simulink model "1"  (R2021a)
settings: Solver=VariableStepAuto  StartTime=0.0  StopTime=3  RelTol=1e-3
libraries: spsThreePhaseVIMeasurementLib x10, spsThreePhaseBreakerLib x9, spsThreePhaseSeriesRLCLoadLib x4, spsThreePhaseTransformerTwoWindingsLib x3, spsRMSLib x2, spsThreePhaseFaultLib x1, spsThreePhaseSourceLib x1, spspowerguiLib x1
settings Model: Creator=ranja  LastModifiedBy=vande

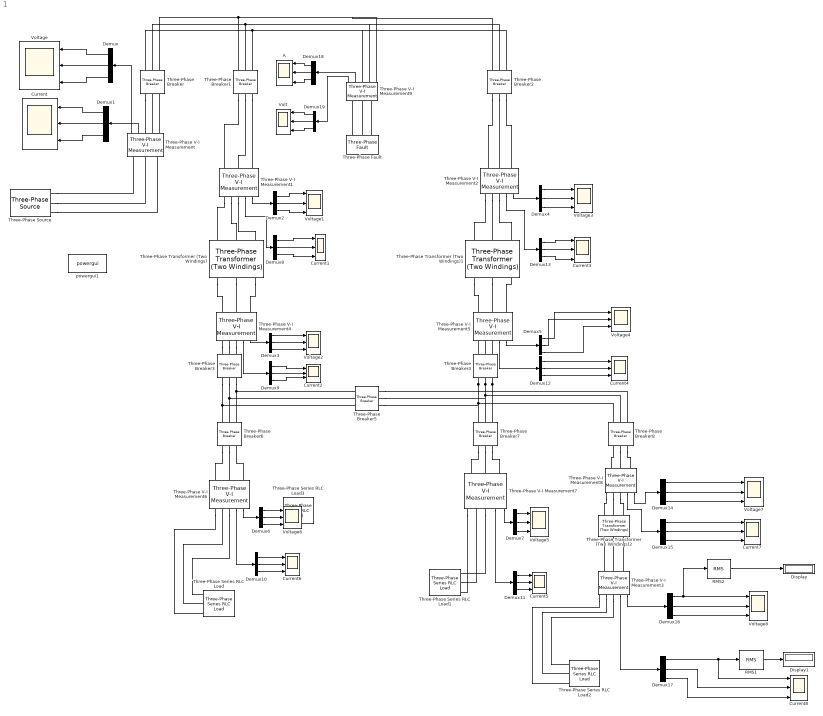
== system 1 ==
  A : Scope  NumInputPorts=3
  Current{,1..8} (9 alike) : Scope  NumInputPorts=3
  Demux{,1..19} (20 alike) : Demux  Outputs=3
  Display : Display
  Display1 : Display
  RMS1 : spsRMSLib/RMS  TrueRMS=on  Freq=50  RMSInit=0  Ts=0
  RMS2 : spsRMSLib/RMS  TrueRMS=on  Freq=50  RMSInit=0  Ts=0
  Three-Phase Series RLC Load : spsThreePhaseSeriesRLCLoadLib/Three-Phase Series RLC Load  LConnTagsString=A|B|C  Configuration=Y (grounded)  NominalVoltage=11e3  Vabc=[1e3 1e3 1e3]  Vabcp=[1e3 1e3 1e3]  NominalFrequency=50  UnbalancedPower=off  ActivePower=500e3  InductivePower=100  CapacitivePower=100  Pabc=[10e3 9e3 11e3]  QLabc=[100 90 110]  QCabc=[100 90 110]  Pabcp=[10e3 9e3 11e3]  QLabcp=[100 90 110]  QCabcp=[100 90 110]  Measurements=None  LoadType=constant Z
  Three-Phase Series RLC Load1 : spsThreePhaseSeriesRLCLoadLib/Three-Phase Series RLC Load  LConnTagsString=A|B|C  Configuration=Y (grounded)  NominalVoltage=11000  Vabc=[1e3 1e3 1e3]  Vabcp=[1e3 1e3 1e3]  NominalFrequency=50  UnbalancedPower=off  ActivePower=500e3  InductivePower=100  CapacitivePower=100  Pabc=[10e3 9e3 11e3]  QLabc=[100 90 110]  QCabc=[100 90 110]  Pabcp=[10e3 9e3 11e3]  QLabcp=[100 90 110]  QCabcp=[100 90 110]  Measurements=None  LoadType=constant Z
  Three-Phase Series RLC Load2 : spsThreePhaseSeriesRLCLoadLib/Three-Phase Series RLC Load  LConnTagsString=A|B|C  Configuration=Y (grounded)  NominalVoltage=433  Vabc=[1e3 1e3 1e3]  Vabcp=[1e3 1e3 1e3]  NominalFrequency=50  UnbalancedPower=off  ActivePower=10e3  InductivePower=5e3  CapacitivePower=10e3  Pabc=[10e3 9e3 11e3]  QLabc=[100 90 110]  QCabc=[100 90 110]  Pabcp=[10e3 9e3 11e3]  QLabcp=[100 90 110]  QCabcp=[100 90 110]  Measurements=None  LoadType=constant Z
  Three-Phase Series RLC Load3 : spsThreePhaseSeriesRLCLoadLib/Three-Phase Series RLC Load  LConnTagsString=A|B|C  Configuration=Y (grounded)  NominalVoltage=11000  Vabc=[1e3 1e3 1e3]  Vabcp=[1e3 1e3 1e3]  NominalFrequency=50  UnbalancedPower=off  ActivePower=500e3  InductivePower=100  CapacitivePower=100  Pabc=[10e3 9e3 11e3]  QLabc=[100 90 110]  QCabc=[100 90 110]  Pabcp=[10e3 9e3 11e3]  QLabcp=[100 90 110]  QCabcp=[100 90 110]  Measurements=None  LoadType=constant Z
  Three-Phase Transformer (Two Windings) : spsThreePhaseTransformerTwoWindingsLib/Three-Phase Transformer (Two Windings)  Winding1Connection=Yg  Winding2Connection=Yg  CoreType=Three single-phase transformers  SetSaturation=off  Hysteresis=off  DataFile='hysteresis'  SetInitialFlux=off  Measurements=None  UNITS=pu  NominalPower=[ 2000e3 , 50 ]  Winding1=[ 33e3 , 0.002 , 0.08 ]  Winding2=[ 11e3 , 0.002 , 0.08 ]  Rm=500  Lm=500  L0=0.5  Saturation=[ 0,0 ; 0.0024,1.2 ; 1.0,1.52 ]  InitialFluxes=[ 0.8 , -0.8 , 0.7 ]  BreakLoop=off  DiscreteSolver=Trapezoidal iterative  DataType=off  TransfoNumber=1
  Three-Phase Transformer (Two Windings)1 : spsThreePhaseTransformerTwoWindingsLib/Three-Phase Transformer (Two Windings)  Winding1Connection=Yg  Winding2Connection=Yg  CoreType=Three single-phase transformers  SetSaturation=off  Hysteresis=off  DataFile='hysteresis'  SetInitialFlux=off  Measurements=None  UNITS=pu  NominalPower=[ 2000e3 , 50 ]  Winding1=[ 33e3 , 0.002 , 0.08 ]  Winding2=[ 11e3 , 0.002 , 0.08 ]  Rm=500  Lm=500  L0=0.5  Saturation=[ 0,0 ; 0.0024,1.2 ; 1.0,1.52 ]  InitialFluxes=[ 0.8 , -0.8 , 0.7 ]  BreakLoop=off  DiscreteSolver=Trapezoidal iterative  DataType=off  TransfoNumber=1
  Three-Phase Transformer (Two Windings)2 : spsThreePhaseTransformerTwoWindingsLib/Three-Phase Transformer (Two Windings)  Winding1Connection=Yg  Winding2Connection=Yg  CoreType=Three single-phase transformers  SetSaturation=off  Hysteresis=off  DataFile='hysteresis'  SetInitialFlux=off  Measurements=None  UNITS=pu  NominalPower=[ 500e3 , 50 ]  Winding1=[ 11e3 , 0.002 , 0.08 ]  Winding2=[ 0.433e3 , 0.002 , 0.08 ]  Rm=500  Lm=500  L0=0.5  Saturation=[ 0,0 ; 0.0024,1.2 ; 1.0,1.52 ]  InitialFluxes=[ 0.8 , -0.8 , 0.7 ]  BreakLoop=off  DiscreteSolver=Trapezoidal iterative  DataType=off  TransfoNumber=1
  Three-Phase V-I Measurement{,1..9} (10 alike) : spsThreePhaseVIMeasurementLib/Three-Phase V-I Measurement  VoltageMeasurement=phase-to-ground  SetLabelV=off  LabelV=Vabc  Vpu=off  VpuLL=off  CurrentMeasurement=yes  SetLabelI=off  LabelI=Iabc  Ipu=off  Pbase=100e6  Vbase=500e3  OutputType=Complex  PhasorSimulation=off  PSBequivalent=0
  Three-Phase Breaker{,1..8} (9 alike) : spsThreePhaseBreakerLib/Three-Phase Breaker  InitialState=closed  SwitchA=on  SwitchB=on  SwitchC=on  SwitchTimes="[1/60  5/60]"  External=off  BreakerResistance=0.01  SnubberResistance=1e6  SnubberCapacitance=inf  Measurements=None
  Three-Phase Fault : spsThreePhaseFaultLib/Three-Phase Fault  InitialStates=0  FaultA=on  FaultB=on  FaultC=on  GroundFault=on  SwitchTimes=[1 1.5]  External=off  SwitchStatus=NaN  FaultResistance=17  GroundResistance=0.01  SnubberResistance=1e6  SnubberCapacitance=inf  Measurements=None
  Three-Phase Source : spsThreePhaseSourceLib/Three-Phase Source  InternalConnection=Yg  VoltagePhases=off  Voltage=33e3  PhaseAngle=0  Voltage_phases=[25e3 25e3 25e3]/sqrt(3)  PhaseAngles_phases=[0 -120 +120]  Frequency=50  NonIdealSource=on  SpecifyImpedance=off  Resistance=0.8929  Inductance=16.58e-3  ShortCircuitLevel=100e6  BaseVoltage=25e3  XRratio=7  BusType=swing  Pref=10e3  Qref=0  Prefabc=[10e3, 10e3, 10e3]  Qrefabc=[0, 0, 0]  Qmin=-inf  Qmax=inf
  Volt : Scope  NumInputPorts=3
  Voltage{,1..8} (9 alike) : Scope  NumInputPorts=3
  powergui1 : spspowerguiLib/powergui  Priority=1  SimulationMode=Discrete  SampleTime=1e-4  frequency=60  Iterations=50  frequencyindice=0  Pbase=100e6  ErrMax=1e-4  UnitsV=kV  UnitsW=MW  buscounter=0  FunctionMessages=off  echomessages=off  EnableUseOfTLC=off  CurrentSourceSwitches=off  DisableSnubberDevices=off  DisableRonSwitches=off  DisableVfSwitches=off  DisplayEquations=off  AutomaticDiscreteSolvers=off  SolverType=Tustin/Backward Euler (TBE)  Interpol=off  ExternalGateDelay=off  methode=off  Ts=100  x0status=blocks  SPID=on  SwTol=0  HookPort=off  NonlinearTolerance=1e-4  nMaxIteration=100  ContinueOnMaxIteration=off  RestoreLinks=warning  ResistiveCurrentMeasurement=off  Frange=[0:2:500]  Ylog=off  Xlog=on  ShowGrid=off  save=off  variable=ZData  structure=0  ZoomFFT=off  StartTime=0.0  cycles=1  DisplayStyle=1  fundamental=60  FreqAxis=off  MaxFrequency=1000  frequencyindicesteady=1  RmsSteady=1  display=off
  wires:
  Three-Phase V-I Measurement/2 -> Demux1/1
  Demux/1 -> Voltage/1
  Demux/3 -> Voltage/3
  Demux/2 -> Voltage/2
  Demux13/3 -> Current3/3
  Demux16/1 -> Voltage8/1, RMS2/1
  Demux1/3 -> Current/3
  Demux16/3 -> Voltage8/3
  RMS1/1 -> Display1/1
  Three-Phase V-I Measurement5/2 -> Demux12/1
  Demux17/3 -> Current8/3
  Demux9/1 -> Current2/1
  Three-Phase V-I Measurement3/1 -> Demux16/1
  Demux17/2 -> Current8/2
  RMS2/1 -> Display/1
  Demux15/2 -> Current7/2
  Three-Phase V-I Measurement/1 -> Demux/1
  Demux14/2 -> Voltage7/2
  Three-Phase V-I Measurement8/1 -> Demux14/1
  Three-Phase V-I Measurement8/2 -> Demux15/1
  Three-Phase V-I Measurement2/2 -> Demux13/1
  Three-Phase V-I Measurement3/2 -> Demux17/1
  Demux13/2 -> Current3/2
  Three-Phase V-I Measurement7/2 -> Demux11/1
  Three-Phase V-I Measurement5/1 -> Demux5/1
  Demux4/3 -> Voltage3/3
  Demux4/2 -> Voltage3/2
  Three-Phase V-I Measurement2/1 -> Demux4/1
  Demux3/3 -> Voltage2/3
  Demux2/2 -> Voltage1/2
  Demux14/1 -> Voltage7/1
  Demux2/1 -> Voltage1/1
  Demux1/2 -> Current/2
  Demux2/3 -> Voltage1/3
  Demux13/1 -> Current3/1
  Demux12/3 -> Current4/3
  Three-Phase V-I Measurement1/1 -> Demux2/1
  Demux11/2 -> Current5/2
  Demux10/3 -> Current6/3
  Demux12/1 -> Current4/1
  Three-Phase V-I Measurement6/2 -> Demux10/1
  Demux11/3 -> Current5/3
  Demux3/1 -> Voltage2/1
  Demux9/3 -> Current2/3
  Demux15/3 -> Current7/3
  Demux10/1 -> Current6/1
  Demux3/2 -> Voltage2/2
  Three-Phase V-I Measurement6/1 -> Demux6/1
  Demux5/2 -> Voltage4/2
  Three-Phase V-I Measurement7/1 -> Demux7/1
  Demux9/2 -> Current2/2
  Demux7/2 -> Voltage5/2
  Demux7/1 -> Voltage5/1
  Demux8/2 -> Current1/2
  Demux11/1 -> Current5/1
  Demux5/3 -> Voltage4/3
  Demux14/3 -> Voltage7/3
  Demux5/1 -> Voltage4/1
  Demux8/3 -> Current1/3
  Demux6/2 -> Voltage6/2
  Demux17/1 -> RMS1/1, Current8/1
  Demux1/1 -> Current/1
  Demux16/2 -> Voltage8/2
  Demux15/1 -> Current7/1
  Demux12/2 -> Current4/2
  Demux4/1 -> Voltage3/1
  Demux7/3 -> Voltage5/3
  Demux6/3 -> Voltage6/3
  Three-Phase V-I Measurement4/2 -> Demux9/1
  Demux10/2 -> Current6/2
  Three-Phase V-I Measurement1/2 -> Demux8/1
  Demux6/1 -> Voltage6/1
  Demux8/1 -> Current1/1
  Three-Phase V-I Measurement4/1 -> Demux3/1
  Three-Phase V-I Measurement9/1 -> Demux19/1
  Three-Phase V-I Measurement9/2 -> Demux18/1
  Demux18/2 -> A/2
  Demux18/1 -> A/1
  Demux18/3 -> A/3
  Demux19/1 -> Volt/1
  Demux19/2 -> Volt/2
  Demux19/3 -> Volt/3
  connections:
  Three-Phase Breaker3/RConn3 -- Three-Phase Breaker5/LConn3 -- Three-Phase Breaker6/LConn3
  Three-Phase Breaker4/RConn2 -- Three-Phase Breaker5/RConn2 -- Three-Phase Breaker7/LConn2 -- Three-Phase Breaker8/LConn2
  Three-Phase Breaker1/LConn3 -- Three-Phase V-I Measurement9/RConn3 -- Three-Phase Breaker2/LConn3 -- Three-Phase Breaker/RConn3
  Three-Phase Breaker3/RConn2 -- Three-Phase Breaker5/LConn2 -- Three-Phase Breaker6/LConn2
  Three-Phase Breaker4/RConn3 -- Three-Phase Breaker5/RConn3 -- Three-Phase Breaker7/LConn3 -- Three-Phase Breaker8/LConn3
  Three-Phase Breaker1/LConn1 -- Three-Phase V-I Measurement9/RConn1 -- Three-Phase Breaker2/LConn1 -- Three-Phase Breaker/RConn1
  Three-Phase Breaker4/RConn1 -- Three-Phase Breaker5/RConn1 -- Three-Phase Breaker8/LConn1 -- Three-Phase Breaker7/LConn1
  Three-Phase Breaker3/RConn1 -- Three-Phase Breaker5/LConn1 -- Three-Phase Breaker6/LConn1
  Three-Phase Breaker1/LConn2 -- Three-Phase V-I Measurement9/RConn2 -- Three-Phase Breaker2/LConn2 -- Three-Phase Breaker/RConn2
  Three-Phase Source/RConn1 -- Three-Phase V-I Measurement/LConn1
  Three-Phase V-I Measurement4/RConn2 -- Three-Phase Breaker3/LConn2
  Three-Phase V-I Measurement/RConn3 -- Three-Phase Breaker/LConn3
  Three-Phase Breaker/LConn1 -- Three-Phase V-I Measurement/RConn1
  Three-Phase V-I Measurement3/RConn1 -- Three-Phase Series RLC Load2/LConn1
  Three-Phase V-I Measurement8/RConn3 -- Three-Phase Transformer (Two Windings)2/LConn3
  Three-Phase Source/RConn3 -- Three-Phase V-I Measurement/LConn3
  Three-Phase Breaker7/RConn3 -- Three-Phase V-I Measurement7/LConn3
  Three-Phase V-I Measurement8/LConn3 -- Three-Phase Breaker8/RConn3
  Three-Phase Breaker2/RConn3 -- Three-Phase V-I Measurement2/LConn3
  Three-Phase Breaker2/RConn1 -- Three-Phase V-I Measurement2/LConn1
  Three-Phase V-I Measurement6/LConn1 -- Three-Phase Breaker6/RConn1
  Three-Phase V-I Measurement1/RConn2 -- Three-Phase Transformer (Two Windings)/LConn2
  Three-Phase Breaker8/RConn2 -- Three-Phase V-I Measurement8/LConn2
  Three-Phase Transformer (Two Windings)/RConn2 -- Three-Phase V-I Measurement4/LConn2
  Three-Phase V-I Measurement2/RConn2 -- Three-Phase Transformer (Two Windings)1/LConn2
  Three-Phase Breaker2/RConn2 -- Three-Phase V-I Measurement2/LConn2
  Three-Phase V-I Measurement3/RConn3 -- Three-Phase Series RLC Load2/LConn3
  Three-Phase V-I Measurement4/RConn3 -- Three-Phase Breaker3/LConn3
  Three-Phase Series RLC Load2/LConn2 -- Three-Phase V-I Measurement3/RConn2
  Three-Phase Breaker8/RConn1 -- Three-Phase V-I Measurement8/LConn1
  Three-Phase Breaker1/RConn1 -- Three-Phase V-I Measurement1/LConn1
  Three-Phase V-I Measurement3/LConn3 -- Three-Phase Transformer (Two Windings)2/RConn3
  Three-Phase V-I Measurement6/RConn3 -- Three-Phase Series RLC Load/LConn3
  Three-Phase V-I Measurement4/RConn1 -- Three-Phase Breaker3/LConn1
  Three-Phase Series RLC Load/LConn2 -- Three-Phase V-I Measurement6/RConn2
  Three-Phase Transformer (Two Windings)/RConn3 -- Three-Phase V-I Measurement4/LConn3
  Three-Phase V-I Measurement2/RConn1 -- Three-Phase Transformer (Two Windings)1/LConn1
  Three-Phase Series RLC Load1/LConn2 -- Three-Phase V-I Measurement7/RConn2
  Three-Phase V-I Measurement7/RConn1 -- Three-Phase Series RLC Load1/LConn1
  Three-Phase Transformer (Two Windings)/RConn1 -- Three-Phase V-I Measurement4/LConn1
  Three-Phase V-I Measurement2/RConn3 -- Three-Phase Transformer (Two Windings)1/LConn3
  Three-Phase V-I Measurement6/RConn1 -- Three-Phase Series RLC Load/LConn1
  Three-Phase Source/RConn2 -- Three-Phase V-I Measurement/LConn2
  Three-Phase V-I Measurement3/LConn2 -- Three-Phase Transformer (Two Windings)2/RConn2
  Three-Phase Breaker4/LConn3 -- Three-Phase V-I Measurement5/RConn3
  Three-Phase Breaker6/RConn2 -- Three-Phase V-I Measurement6/LConn2
  Three-Phase V-I Measurement1/RConn3 -- Three-Phase Transformer (Two Windings)/LConn3
  Three-Phase Transformer (Two Windings)1/RConn1 -- Three-Phase V-I Measurement5/LConn1
  Three-Phase Breaker4/LConn1 -- Three-Phase V-I Measurement5/RConn1
  Three-Phase Breaker1/RConn2 -- Three-Phase V-I Measurement1/LConn2
  Three-Phase Breaker7/RConn1 -- Three-Phase V-I Measurement7/LConn1
  Three-Phase V-I Measurement3/LConn1 -- Three-Phase Transformer (Two Windings)2/RConn1
  Three-Phase V-I Measurement8/RConn2 -- Three-Phase Transformer (Two Windings)2/LConn2
  Three-Phase V-I Measurement7/RConn3 -- Three-Phase Series RLC Load1/LConn3
  Three-Phase V-I Measurement/RConn2 -- Three-Phase Breaker/LConn2
  Three-Phase Breaker7/RConn2 -- Three-Phase V-I Measurement7/LConn2
  Three-Phase Breaker1/RConn3 -- Three-Phase V-I Measurement1/LConn3
  Three-Phase V-I Measurement8/RConn1 -- Three-Phase Transformer (Two Windings)2/LConn1
  Three-Phase Transformer (Two Windings)1/RConn2 -- Three-Phase V-I Measurement5/LConn2
  Three-Phase V-I Measurement1/RConn1 -- Three-Phase Transformer (Two Windings)/LConn1
  Three-Phase Breaker4/LConn2 -- Three-Phase V-I Measurement5/RConn2
  Three-Phase Transformer (Two Windings)1/RConn3 -- Three-Phase V-I Measurement5/LConn3
  Three-Phase Breaker6/RConn3 -- Three-Phase V-I Measurement6/LConn3
  Three-Phase Fault/LConn1 -- Three-Phase V-I Measurement9/LConn1
  Three-Phase Fault/LConn2 -- Three-Phase V-I Measurement9/LConn2
  Three-Phase Fault/LConn3 -- Three-Phase V-I Measurement9/LConn3
